simulink model "PTC_MBDS_Interval_Sample"  (R2013a)
settings: Solver=FixedStepDiscrete  StartTime=0.0  StopTime=100  FixedStep=Auto  RelTol=1e-3
undefined symbols (not defined in the file): MN, MX, sigbuilder_block
libraries: simulink_extras x1, PTC_MBDS_LIB x1
settings Model: Creator=uidl7367  LastModifiedBy=sundeep.tuteja
settings DataIOCC: SignalLoggingSaveFormat=ModelDataLogs
settings OptimizationCC: ExpressionDepthLimit=2147483647  InitFltsAndDblsToZero=on
settings DebuggingCC: SaveWithParameterizedLinksMsg=none  SignalResolutionControl=TryResolveAllWithWarning  SolverPrmCheckMsg=none  InheritedTsInSrcMsg=none  MultiTaskDSMMsg=warning  MultiTaskCondExecSysMsg=none  FcnCallInpInsideContextMsg=UseLocalSettings  StrictBusMsg=Warning
settings RTWCC: IncludeERTFirstTime=on
settings GRTTargetCC: TargetFcnLib=ansi_tfl_tmw.mat  CombineOutputUpdateFcns=off  GRTInterface=on

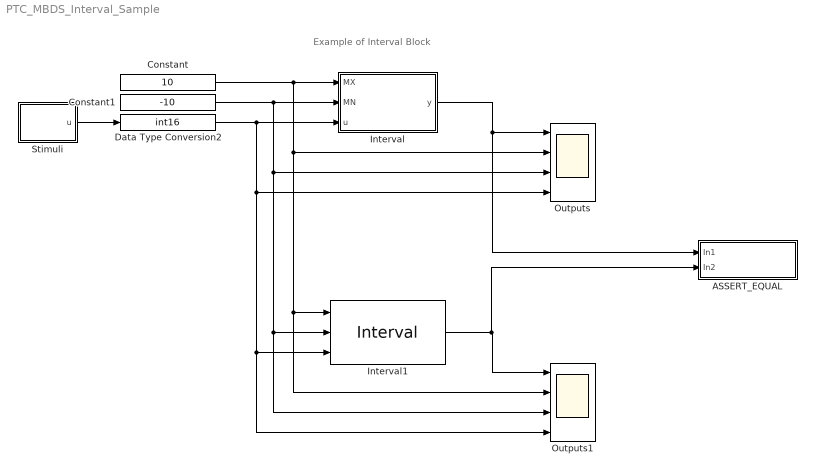
== system PTC_MBDS_Interval_Sample ==
  note: Example of Interval Block
  ASSERT_EQUAL : Subsystem
  Constant : Constant  InitFcn=|  Value=10  OutDataTypeStr=Inherit: Inherit via back propagation
      | if(exist('MBDS_BlockCallback', 'file'))
      |    MBDS_BlockCallback('Update', gcb);  
      | end
  Constant1 : Constant  InitFcn=|  Value=-10  OutDataTypeStr=Inherit: Inherit via back propagation
      | if(exist('MBDS_BlockCallback', 'file'))
      |    MBDS_BlockCallback('Update', gcb);  
      | end
  Data Type Conversion2 : DataTypeConversion  InitFcn=|  OutDataTypeStr=int16  SaturateOnIntegerOverflow=on
      | try
      |    MBDS_BlockCallback('Update', gcb);
      | end
  Interval : Subsystem  InitFcn=|  mask(Interval){MBDS_LibraryBlock=on, IntervalMode=[MN;MX], InputSameDT=on, MBDS_BlockVersion=05.40}
      | if(exist('MBDS_BlockCallback', 'file'))
      |    MBDS_BlockCallback('Update', gcb);
      | end
      mask prompts: MBDS_LibraryBlock "MBDS library block"; IntervalMode "Mode of Operation"; InputSameDT "Require all inputs have the same data"; MBDS_BlockVersion "Block version:"
      mask help: Output is true if u meets the selected Mode of operation for the interval function
      mask init:
      | if(exist('MBDS_BlockCallback', 'file'))
      |    MBDS_BlockCallback('Init', gcb);
      | else
      |    % Disable all mask parameters
      |    MaskEnables = get_param(gcb, 'MaskEnables');
      |    for k = [1:length(MaskEnables)]
      |       MaskEnables{k} = 'off';
      |    end
      |    if(~isequal(MaskEnables, get_param(gcb, 'MaskEnables')))
      |       set_param(gcb, 'MaskEnables', MaskEnables);
      |    end
      | end
      mask Help: eval(['open([workdir(''library_dir:''),''\Blockset\help\'',get_param(gcb,''MaskType''),''.html''])'])
      mask TypeOptions IntervalMode: [MN;MX] | [MN;MX[ | ]MN;MX] | ]MN;MX[
      mask Callback IntervalMode:
      | % Adopt value
      | if(exist('MBDS_BlockCallback', 'file'))
      |    MBDS_BlockCallback('IntervalMode', gcb);
      | end
      mask Display:
      | % Show icon or block text
      | disp(IntervalMode);
      | 
      | % Display port labels
      | port_label('input', 1, 'MX');
      | port_label('input', 2, 'MN');
      | port_label('input', 3, 'u');
      | port_label('output', 1, 'y');
  Interval1 : PTC_MBDS_LIB/MBDS Standard Library/Basic Operations/Logic and Bit Operations/Interval  IntervalMode=[MN;MX]  InputSameDT=on  PTC_MBDS_BlockVersion=5.32  PTC_BlockType=PTC_MBDS_Interval
  Outputs : Scope  NumInputPorts=4
      settings: TimeRange=10  YMin=0~9~-11~-50  YMax=1~11~-9~50  SampleInput=on  SampleTime=1
  Outputs1 : Scope  NumInputPorts=4
      settings: TimeRange=10  YMin=0~9~-11~-50  YMax=1~11~-9~50  SampleInput=on  SampleTime=1
  Stimuli : Subsystem  Tag=STV Subsys  LoadFcn=sigbuilder_block('load');  StartFcn=sigbuilder_block('start');  StopFcn=sigbuilder_block('stop');  ClipboardFcn=sigbuilder_block('clipboard');  mask(Sigbuilder block){}
      mask help: Sigbuilder GUI
      mask init:
      | if ~strcmp(get_param(bdroot(gcb),'SimulationStatus'),'stopped') tuvar = sigbuilder_block('maskInit'); end
      settings: CopyFcn=sigbuilder_block('copy');  DeleteFcn=sigbuilder_block('delete');  ModelCloseFcn=sigbuilder_block('modelClose');  PreSaveFcn=sigbuilder_block('preSave');  PauseFcn=sigbuilder_block('pause')  ContinueFcn=sigbuilder_block('continue')  NameChangeFcn=sigbuilder_block('namechange');  OpenFcn=sigbuilder_block('open',[98.25 121.5 470.25 423.75 ]);  CloseFcn=sigbuilder_block('close');
      mask Display: plot(0,0,100,100,[10,10,40,40,10],[80,20,20,80,80],[40,10],[50,50], [40,27,10],[65,72,56],[40,25,25,10],[28,28,43,43]);
  wires:
  Constant1/1 -> Interval/2(MN), Interval1/2, Outputs1/3, Outputs/3
  Constant/1 -> Interval/1(MX), Interval1/1, Outputs1/2, Outputs/2
  Interval/1(y) -> ASSERT_EQUAL/1(In1), Outputs/1
  Stimuli/1(u) -> Data Type Conversion2/1
  Data Type Conversion2/1 -> Interval/3(u), Interval1/3, Outputs1/4, Outputs/4
  Interval1/1 -> ASSERT_EQUAL/2(In2), Outputs1/1

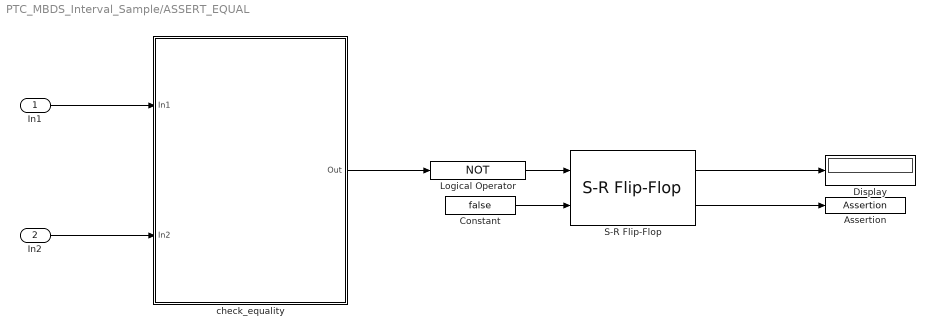
== system PTC_MBDS_Interval_Sample/ASSERT_EQUAL ==
  In1 : Inport
  In2 : Inport  Port=2
  Assertion : Assertion
  Constant : Constant  Value=false
  Display : Display
  Logical Operator : Logic  Operator=NOT  AllPortsSameDT=off  OutDataTypeStr=boolean
  S-R Flip-Flop : simulink_extras/Flip Flops/S-R Flip-Flop  initial_condition=0
  check_equality : MATLAB Function  TreatAsAtomicUnit=on
  wires:
  S-R Flip-Flop/1 -> Display/1
  check_equality/1(Out) -> Logical Operator/1
  Constant/1 -> S-R Flip-Flop/2
  S-R Flip-Flop/2 -> Assertion/1
  In2/1 -> check_equality/2(In2)
  In1/1 -> check_equality/1(In1)
  Logical Operator/1 -> S-R Flip-Flop/1

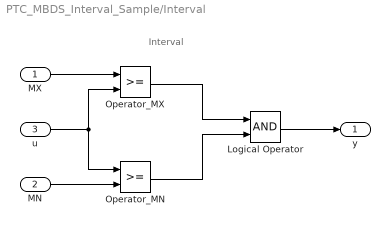
== system PTC_MBDS_Interval_Sample/Interval ==
  note: Interval
  MX : Inport
  MN : Inport  Port=2
  u : Inport  Port=3
  Logical Operator : Logic  AllPortsSameDT=off  OutDataTypeStr=boolean
  Operator_MN : RelationalOperator  OutDataTypeStr=boolean  InputSameDT=on
  Operator_MX : RelationalOperator  OutDataTypeStr=boolean  InputSameDT=on
  y : Outport
  wires:
  MX/1 -> Operator_MX/1
  Operator_MN/1 -> Logical Operator/2
  Operator_MX/1 -> Logical Operator/1
  Logical Operator/1 -> y/1
  u/1 -> Operator_MX/2, Operator_MN/1
  MN/1 -> Operator_MN/2

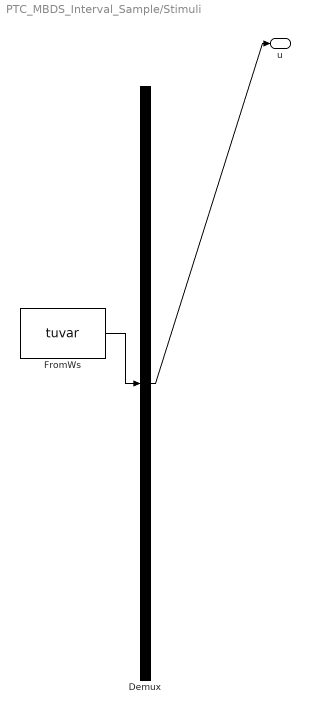
== system PTC_MBDS_Interval_Sample/Stimuli ==
  Demux : Demux  Tag=STV Demux  Outputs=1
  FromWs : FromWorkspace  Tag=STV FromWs  VariableName=tuvar  SampleTime=1  OutputAfterFinalValue=Holding final value
      SigBuilderData=|
      | common.afterFinalStr = 'Hold final value'
      | common.sampleTime = 1
      | dataSet.timeRange = [0 10]
      | dataSet.name = 'test data'
      | sbobj.Groups.Name = 'test data'
      | sbobj.Groups.Signals.Name = 'u'
      | sbobj.Groups.Signals.XData = [0 10]
      | sbobj.Groups.Signals.YData = [-50 50]
  u : Outport  Tag=STV Outport
  wires:
  FromWs/1 -> Demux/1
  Demux/1 -> u/1

== matlab function PTC_MBDS_Interval_Sample/ASSERT_EQUAL/check_equality ==
  data: In1 input; Out output; In2 input
function Out = check_equality(In1, In2)
%#codegen

Out = isequaln(In1, In2);

end
